simulink model "problem2"  (R2019b)
settings: Solver=VariableStepAuto  StartTime=0.0  StopTime=10.0  RelTol=1e-3
settings Model: Creator=davis  LastModifiedBy=davis

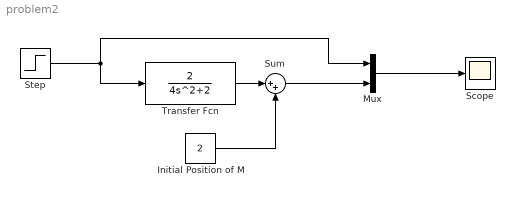
== system problem2 ==
  Initial Position of M : Constant  Value=2
  Mux : Mux  Inputs=2
  Scope : Scope
  Step : Step  Time=0  After=4  SampleTime=0
  Sum : Sum  Inputs=|++
  Transfer Fcn : TransferFcn  Numerator=[2]  Denominator=[4 0 2]
  wires:
  Mux/1 -> Scope/1
  Transfer Fcn/1 -> Sum/1
  Initial Position of M/1 -> Sum/2
  Sum/1 -> Mux/2
  Step/1 -> Transfer Fcn/1, Mux/1
